simulink model "ex4pdimp"  (R2025b)
settings: Solver=VariableStepAuto  StartTime=0.0  StopTime=353  RelTol=1e-3
values from neighbouring files (symbols this model uses):
  IJ = inv(J)    [ex1slidingmode.m]    (also in ex4pdcon.m)
  J = diag([10400, 8200, 9200])    [ex1slidingmode.m]    (also in ex4pdcon.m = diag([7300, 7000, 3800]))
  q0 = [0.68438 ... (first row only)    [ex1slidingmode.m]    (also in ex4pdcon.m = [1;0;0;0])
  qr = [0;1;0;0]    [ex1slidingmode.m]    (also in ex4pdcon.m = [-0.57352)
  w0 = [0;0;0]    [ex1slidingmode.m]    (also in ex4pdcon.m)
libraries: vrlib x1
settings Model: Creator=Esteban  LastModifiedBy=Esteban

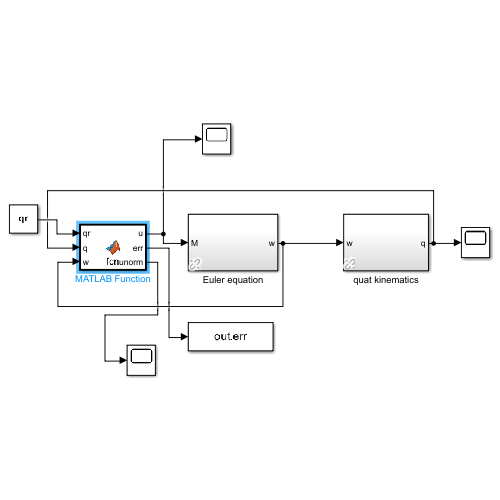
[thumbnail: Simulink's stored preview of the top-level diagram]
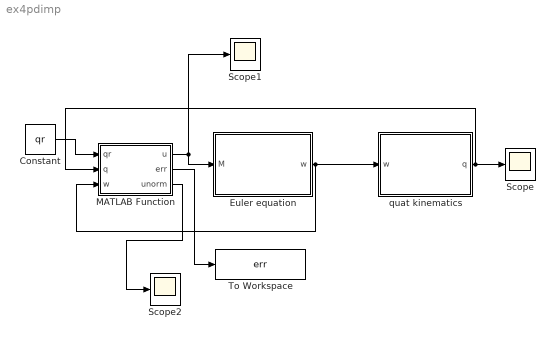
== system ex4pdimp ==
  Constant : Constant  Value=qr
  Euler equation : Subsystem  AncestorBlock=lib_rotations_2014/Euler equation
  MATLAB Function : MATLAB Function  TreatAsAtomicUnit=on
  Scope : Scope
  Scope1 : Scope
      settings: ActiveDisplayYMinimum=-29.03844905695162  ActiveDisplayYMaximum=48.04714020173239
  Scope2 : Scope
      settings: ActiveDisplayYMinimum=-11.350989929511307  ActiveDisplayYMaximum=233.33162152697594  DataLoggingVariableName=ScopeData2
  To Workspace : ToWorkspace  VariableName=err  SaveFormat=Timeseries  SampleTime=-1
  quat kinematics : Subsystem  AncestorBlock=lib_rotations_2014/quat kinematics
  wires:
  Euler equation/1(w) -> MATLAB Function/3(w), quat kinematics/1(w)
  Constant/1 -> MATLAB Function/1(qr)
  MATLAB Function/1(u) -> Euler equation/1(M), Scope1/1
  quat kinematics/1(q) -> MATLAB Function/2(q), Scope/1
  MATLAB Function/2(err) -> To Workspace/1
  MATLAB Function/3(unorm) -> Scope2/1

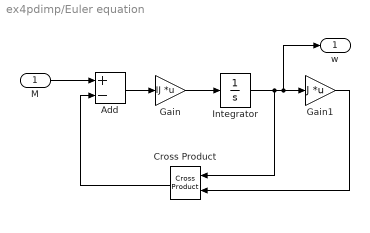
== system ex4pdimp/Euler equation ==
  M : Inport
  Add : Sum  Inputs=+-
  Cross Product : vrlib/Utilities/Cross Product
  Gain : Gain  Gain=IJ  Multiplication=Matrix(K*u)
  Gain1 : Gain  Gain=J  Multiplication=Matrix(K*u)
  Integrator : Integrator  InitialCondition=w0
  w : Outport  VectorParamsAs1DForOutWhenUnconnected=off
  wires:
  Cross Product/1 -> Add/2
  Add/1 -> Gain/1
  Gain1/1 -> Cross Product/2
  Gain/1 -> Integrator/1
  Integrator/1 -> Gain1/1, w/1, Cross Product/1
  M/1 -> Add/1

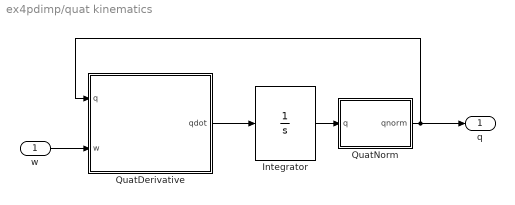
== system ex4pdimp/quat kinematics ==
  w : Inport  PortDimensions=3
  Integrator : Integrator  InitialCondition=q0
  QuatDerivative : MATLAB Function  TreatAsAtomicUnit=on
  QuatNorm : MATLAB Function  TreatAsAtomicUnit=on
  q : Outport  PortDimensions=4  VectorParamsAs1DForOutWhenUnconnected=off
  wires:
  w/1 -> QuatDerivative/2(w)
  QuatDerivative/1(qdot) -> Integrator/1
  QuatNorm/1(qnorm) -> QuatDerivative/1(q), q/1
  Integrator/1 -> QuatNorm/1(q)

== matlab function ex4pdimp/quat kinematics/QuatDerivative ==
  data: q input; qdot output; w input
function qdot= QuatDerivative(q,w)
%#codegen
omegaq=[0; w];
Q=[q(1) -q(2) -q(3) -q(4);
    q(2) q(1) -q(4) q(3);
    q(3) q(4) q(1) -q(2);
    q(4) -q(3) q(2) q(1)];
qdot=Q*omegaq/2;

== matlab function ex4pdimp/quat kinematics/QuatNorm ==
  data: q input; qnorm output
function qnorm = QuatNorm(q)
%#codegen
qnorm=zeros(4,1);
q2=sqrt(q'*q);
qnorm=q/q2;

== matlab function ex4pdimp/MATLAB Function ==
  data: qr input; u output; q input; w input; err output; unorm output
function [u,err,unorm] = fcn(qr,q,w)

k1 = 20;
k2 = 196;

qs = [q(1);-q(2:4)];

dq = quatprod(qs,qr);

dq = dq(2:4);


err = norm(dq);
u = k1*dq - k2*w;

unorm = norm(u);
